simulink model "Robot_Model_new"  (R2021a)
settings: Solver=FixedStepAuto  StartTime=0.0  StopTime=10  FixedStep=Auto  RelTol=1e-3
values from neighbouring files (symbols this model uses):
  Bm = 3.1586e-06    [init.m]
  K = [1 0 0 0;0 1 0 0]    [init.m]
  Ke = 0.00806    [init.m]
  Kt = 0.012    [init.m]
  L = [0;0]    [init.m]
  M = [0 0 1 0;0 0 0 1;-inv(W)*Z -inv(W)*Y]    [init.m]
  N = [0;0;inv(W)*J]    [init.m]
  R = 1.261    [init.m]
libraries: fuzblock x1
settings Model: Creator=ziad  LastModifiedBy=Roy
settings DebuggingCC: SFMachineParentedDataDiag=warning

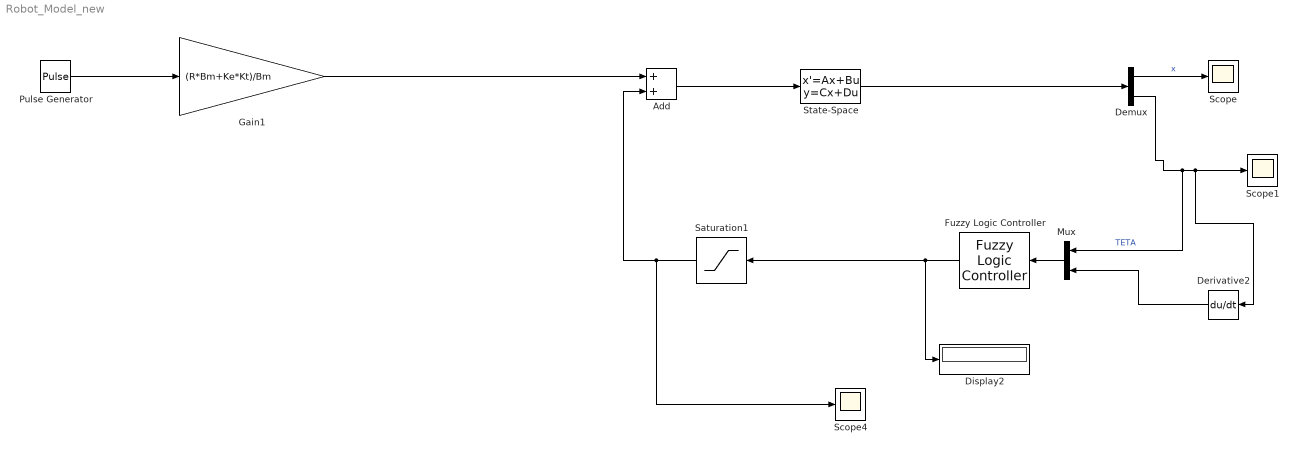
== system Robot_Model_new ==
  Add : Sum
  Demux : Demux  Outputs=2
  Derivative2 : Derivative
  Display2 : Display
  Fuzzy Logic Controller : fuzblock/Fuzzy Logic  Controller  FIS="\"CPFIS_damped5.8.fis\""  OutputSampleNumber=101  DataType=double  FuzzifiedInputs=off  RuleFiringStrengths=off  RuleOutputs=off  AggregatedOutputs=off  SimulateUsing=Interpreted execution  OutOfRangeInputValueMessage=warning  NoRuleFiredMessage=warning  EmptyOutputFuzzySetMessage=warning
  Gain1 : Gain  Gain=(R*Bm+Ke*Kt)/Bm
  Mux : Mux  Inputs=2
  Pulse Generator : DiscretePulseGenerator  PulseType=Time based  Amplitude=0.2  Period=10  PhaseDelay=1
  Saturation1 : Saturate  UpperLimit=7.2  LowerLimit=-7.2
  Scope : Scope
  Scope1 : Scope
  Scope4 : Scope
  State-Space : StateSpace  A=M  B=N  C=K  D=L  InitialCondition=0
  wires:
  Demux/1 -> Scope/1  "x"
  Demux/2 -> Mux/1, Derivative2/1, Scope1/1  "TETA"
  State-Space/1 -> Demux/1
  Pulse Generator/1 -> Gain1/1
  Fuzzy Logic Controller/1 -> Saturation1/1, Display2/1
  Mux/1 -> Fuzzy Logic Controller/1
  Derivative2/1 -> Mux/2
  Saturation1/1 -> Add/2, Scope4/1
  Add/1 -> State-Space/1
  Gain1/1 -> Add/1
